simulink model "Sine_Wave"  (R2024b)
settings: Solver=FixedStepAuto  StartTime=0.0  StopTime=10.0  FixedStep=0.0001  MaxStep=0.001  RelTol=0.001
settings Model: Creator=abdal  LastModifiedBy=abdal

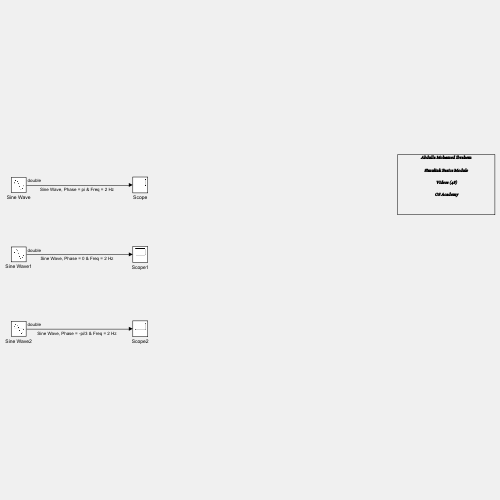
[thumbnail: Simulink's stored preview of the top-level diagram]
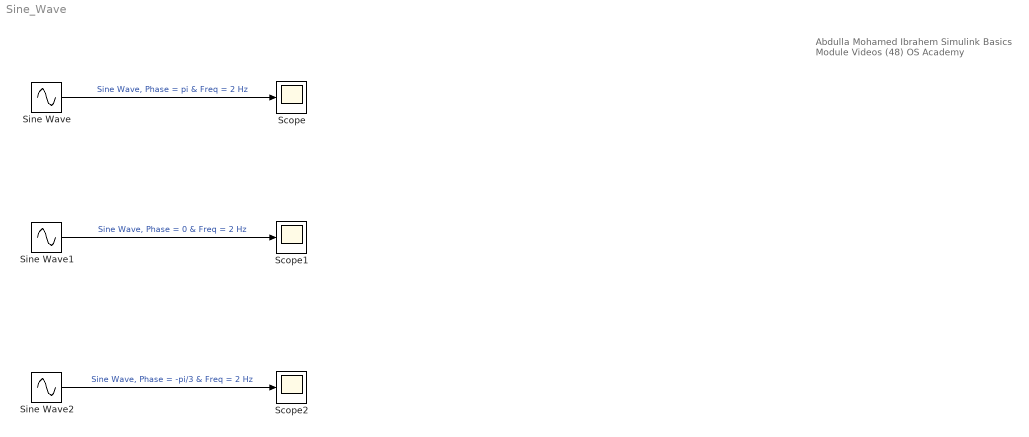
== system Sine_Wave ==
  note: Abdulla Mohamed Ibrahem
      | Simulink Basics Module
      | Videos (48)
      | OS Academy
  Scope : Scope
  Scope1 : Scope
  Scope2 : Scope
  Sine Wave : Sin  Amplitude=5  Frequency=2*pi*2  Phase=pi  SampleTime=0
  Sine Wave1 : Sin  Amplitude=5  Frequency=2*pi*2  SampleTime=0
  Sine Wave2 : Sin  Amplitude=5  Frequency=2*pi*2  Phase=-pi/3  SampleTime=0
  wires:
  Sine Wave/1 -> Scope/1  "Sine Wave, Phase = pi & Freq = 2 Hz"
  Sine Wave1/1 -> Scope1/1  "Sine Wave, Phase = 0 & Freq = 2 Hz"
  Sine Wave2/1 -> Scope2/1  "Sine Wave, Phase = -pi/3 & Freq = 2 Hz"
